simulink model "FOC_PMSM"  (R2021a)
settings: Solver=ode3  StartTime=0.0  StopTime=1  FixedStep=1e-6  RelTol=1e-3
InitFcn:
  | Td=1/5000;
  | Ld=0.0057;
  | Lq=0.0125;
  | r=1.2;
  | P=4;
  | Ld=0.0125;
  | Lq=0.0057;
  | PhiPM=0.123;
  | Vdc=700;
  | B=0;
  | J=0.0027;
  | fs=5000;
libraries: pid_lib x7, spsThreePhaseSeriesRLCBranchLib x3, spsThreePhaseVIMeasurementLib x2, spsdq0toabcLib x2, autolibpmsminterior x1, spsDCVoltageSourceLib x1, spsGroundLib x1, spsSVPWMGenerator2LevelLib x1, spsUniversalBridgeLib x1, spsabctoAlphaBetaZeroLib x1, spspowerguiLib x1, simulink x1
settings Model: Creator=Mostafa  LastModifiedBy=Mostafa

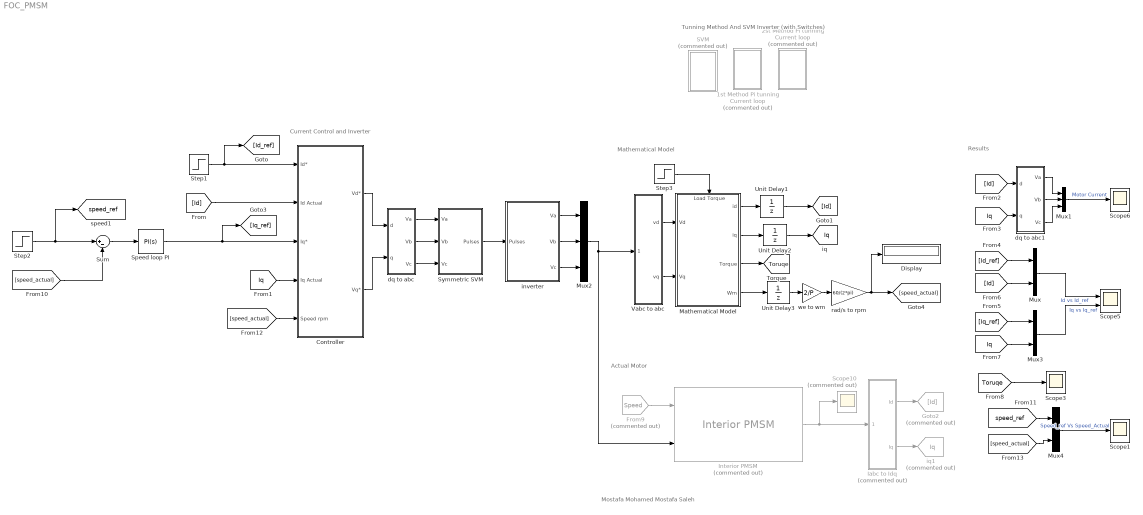
== system FOC_PMSM ==
  note: Tunning Method And SVM Inverter (with Switches)
  note: Current Control and Inverter
  note: Actual Motor
  note: Mathematical Model
  note: Results
  note: Mostafa Mohamed Mostafa Saleh
  1st Method Pi tunning Current loop : Subsystem  Commented=on
  2st Method Pi tunning Current loop : Subsystem  Commented=on
  Controller : Subsystem
  Display : Display
  From9 : From  Commented=on  GotoTag=Speed  TagVisibility=global
  Goto2 : Goto  Commented=on  GotoTag=Id
  Iabc to Idq : Subsystem  Commented=on
  Interior PMSM : autolibpmsminterior/Interior PMSM  Commented=on  port_config=Speed  sim_type=Continuous  Ts=0.001  P=2  Rs=1.2  Ldq=[0.125 0.057]  KConstText=Permanent flux linkage constant (lambda_pm):  lambda_pm=0.123  Ke=159.9771  mechanical=[0.0027, 4.924e-4, 0]  idq0=[0 0]  theta_init=0  omega_init=0  KConst=0.123  lambda_pm_calc=0.123  Kt=1.323  RefBlkName='autolibpmsminterior/Interior PMSM'  aMode=1
      settings: SourceProductBaseCode=PW,MT,VE,VP
  Mathematical Model : Subsystem
      settings: PortSchema="{\"entries\":[{\"content\":{\"sides\":[{\"content\":{\"connectorIds\":[\"In1\",\"In2\"]},\"type\":\"ConnectorPlacement.EquallySpacedRectSide\",\"uuid\":\"051f3cf9-9be1-4106-b38d-66cc7393fb99\"},{\"content\":{\"connectorIds\":[\"Out1\",\"Out2\",\"Out3\",\"Out4\"],\"side\":\"RIGHT\"},\"type\":\"ConnectorPlacement.EquallySpacedRectSide\",\"uuid\":\"0ae6f8d8-defd-4982-a857-4d094ecd69f7\"},{\"content\":{\"connectorIds\":[\"In3\"],\"side\":\"TOP\"},\"type\":\"ConnectorPlacement.EquallySpacedRectSide\",\"uuid\":\"9e822861-0fa2-4e7e-872b-d3c49c871a81\"}]},\"type\":\"ConnectorPlacement.EquallySpacedConnector\",\"uuid\":\"055cbe4c-d848-4a6f-bb15-48a4c380dc2b\"}],\"packageUris\":[\"http://schema.mathworks.com/mf0/Connector/R2020b\"],\"version\":\"1.0\"}"
  Mux : Mux  Inputs=2
  Mux1 : Mux  Inputs=3
  Mux2 : Mux  Inputs=3
  Mux3 : Mux  Inputs=2
  Mux4 : Mux  Inputs=2
  SVM : Subsystem  Commented=on
  Scope1 : Scope
  Scope10 : Scope  Commented=on
  Scope3 : Scope
  Scope5 : Scope  NumInputPorts=2
  Scope6 : Scope
  Speed loop PI : pid_lib/PID Controller  Controller=PI  Form=Parallel  TimeDomain=Continuous-time  UseExternalTs=off  SampleTime=-1  IntegratorMethod=Forward Euler  FilterMethod=Forward Euler  ControllerParametersSource=internal  P=0.642857  I=76.5306  D=0  UseFilter=on  N=100  TunerSelectOption=Transfer Function Based (PID Tuner App)  ZeroCross=off  InitialConditionSource=internal  InitialConditionForIntegrator=0  InitialConditionForFilter=0  DifferentiatorICPrevScaledInput=0  ExternalReset=none  TrackingMode=off  Kt=1  LimitOutput=on  SatLimitsSource=internal  UpperSaturationLimit=20  LowerSaturationLimit=-20  LinearizeAsGain=off  AntiWindupMode=clamping  Kb=1  POutMin=[]  POutMax=[]  IOutMin=[]  IOutMax=[]  DOutMin=[]  DOutMax=[]  NOutMin=[]  NOutMax=[]  SumOutMin=[]  SumOutMax=[]  SaturationOutMin=[]  SaturationOutMax=[]  PParamMin=[]  PParamMax=[]  IParamMin=[]  IParamMax=[]  DParamMin=[]  DParamMax=[]  NParamMin=[]  NParamMax=[]  KbParamMin=[]  KbParamMax=[]  KtParamMin=[]  KtParamMax=[]  KbOutMin=[]  KbOutMax=[]  KtOutMin=[]  KtOutMax=[]  IntegratorOutMin=[]  IntegratorOutMax=[]  FilterOutMin=[]  FilterOutMax=[]  SumI1OutMin=[]  SumI1OutMax=[]  SumI2OutMin=[]  SumI2OutMax=[]  SumI3OutMin=[]  SumI3OutMax=[]  SumI4OutMin=[]  SumI4OutMax=[]  SumDOutMin=[]  SumDOutMax=[]  DifferentiatorOutMin=[]  DifferentiatorOutMax=[]  FilterDiffOutCoefMin=[]  FilterDiffOutCoefMax=[]  ReciprocalOutMin=[]  ReciprocalOutMax=[]  SumDenOutMin=[]  SumDenOutMax=[]  SumNumOutMin=[]  SumNumOutMax=[]  DivideOutMin=[]  DivideOutMax=[]  UdiffTsProdOutMin=[]  UdiffTsProdOutMax=[]  NTsProdOutMin=[]  NTsProdOutMax=[]  UintegralTsProdOutMin=[]  UintegralTsProdOutMax=[]  UngainTsProdOutMin=[]  UngainTsProdOutMax=[]  IntegratorContinuousStateAttributes=''  IntegratorStateMustResolveToSignalObject=off  IntegratorRTWStateStorageClass=Auto  FilterContinuousStateAttributes=''  FilterStateMustResolveToSignalObject=off  FilterRTWStateStorageClass=Auto  ParallelPVariant=InternalParameters  IdealPVariant=Disabled  IVariant=InternalParameters  DVariant=Disabled  IntegratorVariant=Continuous  SatVariant=Enabled  AWVariant=ContClampingParallel  PCopyVariant=Disabled  TRVariant=Disabled  FdbkBlocksVariant=Forward  IdealPFdbkVariant=Disabled  SatFdbkVariant=Disabled  DerivativeFilterVariant=Disabled  NVariant=Disabled  NCopyVariant=Disabled_SignalSpec  FilterICVariant=Disabled  IntegratorICVariant=InternalICs  ExternalResetVariant=Disabled  TRSumVariant=Passthrough  SumFdbkVariant=Disabled  SumVariant=Sum_PI  TsampFilterVariant=InternalTs  TsampNgainVariant=Passthrough  TsampIntegralVariant=Passthrough  ExternalSaturationOutDataTypeStr=Inherit: Same as second input
  Step1 : Step  Time=0.2  After=0  SampleTime=0
  Step2 : Step  Time=0.2  After=1000  SampleTime=0
  Step3 : Step  Time=0.6  After=5  SampleTime=0
  Sum : Sum  Inputs=|+-
  Symmetric SVM : Subsystem
  Unit Delay1 : UnitDelay  SampleTime=-1  HasFrameUpgradeWarning=on
  Unit Delay2 : UnitDelay  SampleTime=-1  HasFrameUpgradeWarning=on
  Unit Delay3 : UnitDelay  SampleTime=-1  HasFrameUpgradeWarning=on
  Vabc to abc : Subsystem
  dq to abc : Subsystem
  dq to abc1 : Subsystem
  inverter : Subsystem
  iq1 : Goto  Commented=on  GotoTag=Iq  TagVisibility=global
  rad/s to rpm : Gain  Gain=60/(2*pi)
  we to wm : Gain  Gain=2/P
  tag scope: Iq=global, Toruqe=global, speed_ref=global
  wires:
  [Id] -> dq to abc1/1(d)
  [Toruqe] -> Scope3/1
  [Iq_ref] -> Mux3/1
  [Id] -> Mux/2
  Mux/1 -> Scope5/1  "Id vs Id_ref"
  Mux3/1 -> Scope5/2  "Iq vs Iq_ref"
  [Iq] -> Mux3/2
  [Id_ref] -> Mux/1
  [Iq] -> dq to abc1/2(q)
  Unit Delay2/1 -> [Iq]
  Step3/1 -> Mathematical Model/3(Load Torque)
  Mathematical Model/4(Wm) -> Unit Delay3/1
  Mathematical Model/2(iq) -> Unit Delay2/1
  Vabc to abc/1(vd) -> Mathematical Model/1(Vd)
  Vabc to abc/2(vq) -> Mathematical Model/2(Vq)
  Mathematical Model/3(Torque) -> [Toruqe]
  Unit Delay1/1 -> [Id]
  Mathematical Model/1(id) -> Unit Delay1/1
  Iabc to Idq/1(Id) -> Goto2/1
  From9/1 -> Interior PMSM/1
  Iabc to Idq/2(Iq) -> iq1/1
  Interior PMSM/2 -> Iabc to Idq/1(Iabc), Scope10/1
  Mux2/1 -> Interior PMSM/2, Vabc to abc/1(Vabc)
  inverter/1(Va) -> Mux2/1
  inverter/2(Vb) -> Mux2/2
  inverter/3(Vc) -> Mux2/3
  [Iq] -> Controller/4("Iq Actual ")
  Speed loop PI/1 -> [Iq_ref], Controller/3(Iq*)
  Symmetric SVM/1(Pulses) -> inverter/1(Pulses)
  dq to abc/1(Va) -> Symmetric SVM/1(Va)
  Controller/2(Vq*) -> dq to abc/2(q)
  dq to abc/2(Vb) -> Symmetric SVM/2(Vb)
  Step1/1 -> Controller/1(Id*), [Id_ref]
  [Id] -> Controller/2("Id Actual ")
  Controller/1(Vd*) -> dq to abc/1(d)
  dq to abc/3(Vc) -> Symmetric SVM/3(Vc)
  dq to abc1/1(Va) -> Mux1/1
  dq to abc1/2(Vb) -> Mux1/2
  dq to abc1/3(Vc) -> Mux1/3
  Mux1/1 -> Scope6/1  "Motor Current"
  Step2/1 -> [speed_ref], Sum/1
  [speed_actual] -> Sum/2
  Sum/1 -> Speed loop PI/1
  [speed_actual] -> Controller/5(Speed rpm)
  we to wm/1 -> rad/s to rpm/1
  Unit Delay3/1 -> we to wm/1
  rad/s to rpm/1 -> [speed_actual], Display/1
  [speed_ref] -> Mux4/1
  [speed_actual] -> Mux4/2
  Mux4/1 -> Scope1/1  "Speed_ref Vs Speed_Actual"

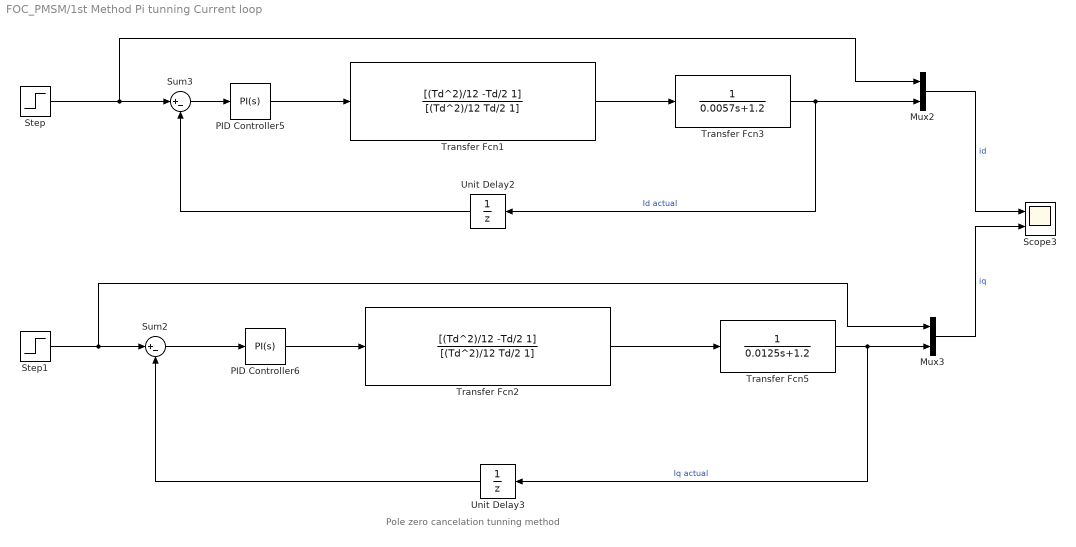
== system FOC_PMSM/1st Method Pi tunning Current loop ==
  note: Pole zero cancelation tunning method
  Mux2 : Mux  Inputs=2
  Mux3 : Mux  Inputs=2
  PID Controller5 : pid_lib/PID Controller  Controller=PI  Form=Parallel  TimeDomain=Continuous-time  UseExternalTs=off  SampleTime=-1  IntegratorMethod=Forward Euler  FilterMethod=Forward Euler  ControllerParametersSource=internal  P=9.405  I=1980  D=0  UseFilter=on  N=100  TunerSelectOption=Transfer Function Based (PID Tuner App)  InitialConditionSource=internal  InitialConditionForIntegrator=0  InitialConditionForFilter=0  DifferentiatorICPrevScaledInput=0  ExternalReset=none  TrackingMode=off  Kt=1  LimitOutput=off  SatLimitsSource=internal  UpperSaturationLimit=inf  LowerSaturationLimit=-inf  LinearizeAsGain=on  AntiWindupMode=clamping  Kb=1  POutMin=[]  POutMax=[]  IOutMin=[]  IOutMax=[]  DOutMin=[]  DOutMax=[]  NOutMin=[]  NOutMax=[]  SumOutMin=[]  SumOutMax=[]  SaturationOutMin=[]  SaturationOutMax=[]  PParamMin=[]  PParamMax=[]  IParamMin=[]  IParamMax=[]  DParamMin=[]  DParamMax=[]  NParamMin=[]  NParamMax=[]  KbParamMin=[]  KbParamMax=[]  KtParamMin=[]  KtParamMax=[]  KbOutMin=[]  KbOutMax=[]  KtOutMin=[]  KtOutMax=[]  IntegratorOutMin=[]  IntegratorOutMax=[]  FilterOutMin=[]  FilterOutMax=[]  SumI1OutMin=[]  SumI1OutMax=[]  SumI2OutMin=[]  SumI2OutMax=[]  SumI3OutMin=[]  SumI3OutMax=[]  SumI4OutMin=[]  SumI4OutMax=[]  SumDOutMin=[]  SumDOutMax=[]  DifferentiatorOutMin=[]  DifferentiatorOutMax=[]  FilterDiffOutCoefMin=[]  FilterDiffOutCoefMax=[]  ReciprocalOutMin=[]  ReciprocalOutMax=[]  SumDenOutMin=[]  SumDenOutMax=[]  SumNumOutMin=[]  SumNumOutMax=[]  DivideOutMin=[]  DivideOutMax=[]  UdiffTsProdOutMin=[]  UdiffTsProdOutMax=[]  NTsProdOutMin=[]  NTsProdOutMax=[]  UintegralTsProdOutMin=[]  UintegralTsProdOutMax=[]  UngainTsProdOutMin=[]  UngainTsProdOutMax=[]  IntegratorContinuousStateAttributes=''  IntegratorStateMustResolveToSignalObject=off  IntegratorRTWStateStorageClass=Auto  FilterContinuousStateAttributes=''  FilterStateMustResolveToSignalObject=off  FilterRTWStateStorageClass=Auto  ParallelPVariant=InternalParameters  IdealPVariant=Disabled  IVariant=InternalParameters  DVariant=Disabled  IntegratorVariant=Continuous  SatVariant=Disabled  AWVariant=Passthrough  PCopyVariant=Disabled  TRVariant=Disabled  FdbkBlocksVariant=Forward  IdealPFdbkVariant=Disabled  SatFdbkVariant=Disabled  DerivativeFilterVariant=Disabled  NVariant=Disabled  NCopyVariant=Disabled_SignalSpec  FilterICVariant=Disabled  IntegratorICVariant=InternalICs  ExternalResetVariant=Disabled  TRSumVariant=Passthrough  SumFdbkVariant=Disabled  SumVariant=Sum_PI  TsampFilterVariant=InternalTs  TsampNgainVariant=Passthrough  TsampIntegralVariant=Passthrough  ExternalSaturationOutDataTypeStr=Inherit: Same as second input
  PID Controller6 : pid_lib/PID Controller  Controller=PI  Form=Parallel  TimeDomain=Continuous-time  UseExternalTs=off  SampleTime=-1  IntegratorMethod=Forward Euler  FilterMethod=Forward Euler  ControllerParametersSource=internal  P=20.625  I=1980  D=0  UseFilter=on  N=100  TunerSelectOption=Transfer Function Based (PID Tuner App)  ZeroCross=off  InitialConditionSource=internal  InitialConditionForIntegrator=0  InitialConditionForFilter=0  DifferentiatorICPrevScaledInput=0  ExternalReset=none  TrackingMode=off  Kt=1  LimitOutput=off  SatLimitsSource=internal  UpperSaturationLimit=inf  LowerSaturationLimit=-inf  LinearizeAsGain=on  AntiWindupMode=clamping  Kb=1  POutMin=[]  POutMax=[]  IOutMin=[]  IOutMax=[]  DOutMin=[]  DOutMax=[]  NOutMin=[]  NOutMax=[]  SumOutMin=[]  SumOutMax=[]  SaturationOutMin=[]  SaturationOutMax=[]  PParamMin=[]  PParamMax=[]  IParamMin=[]  IParamMax=[]  DParamMin=[]  DParamMax=[]  NParamMin=[]  NParamMax=[]  KbParamMin=[]  KbParamMax=[]  KtParamMin=[]  KtParamMax=[]  KbOutMin=[]  KbOutMax=[]  KtOutMin=[]  KtOutMax=[]  IntegratorOutMin=[]  IntegratorOutMax=[]  FilterOutMin=[]  FilterOutMax=[]  SumI1OutMin=[]  SumI1OutMax=[]  SumI2OutMin=[]  SumI2OutMax=[]  SumI3OutMin=[]  SumI3OutMax=[]  SumI4OutMin=[]  SumI4OutMax=[]  SumDOutMin=[]  SumDOutMax=[]  DifferentiatorOutMin=[]  DifferentiatorOutMax=[]  FilterDiffOutCoefMin=[]  FilterDiffOutCoefMax=[]  ReciprocalOutMin=[]  ReciprocalOutMax=[]  SumDenOutMin=[]  SumDenOutMax=[]  SumNumOutMin=[]  SumNumOutMax=[]  DivideOutMin=[]  DivideOutMax=[]  UdiffTsProdOutMin=[]  UdiffTsProdOutMax=[]  NTsProdOutMin=[]  NTsProdOutMax=[]  UintegralTsProdOutMin=[]  UintegralTsProdOutMax=[]  UngainTsProdOutMin=[]  UngainTsProdOutMax=[]  IntegratorContinuousStateAttributes=''  IntegratorStateMustResolveToSignalObject=off  IntegratorRTWStateStorageClass=Auto  FilterContinuousStateAttributes=''  FilterStateMustResolveToSignalObject=off  FilterRTWStateStorageClass=Auto  ParallelPVariant=InternalParameters  IdealPVariant=Disabled  IVariant=InternalParameters  DVariant=Disabled  IntegratorVariant=Continuous  SatVariant=Disabled  AWVariant=Passthrough  PCopyVariant=Disabled  TRVariant=Disabled  FdbkBlocksVariant=Forward  IdealPFdbkVariant=Disabled  SatFdbkVariant=Disabled  DerivativeFilterVariant=Disabled  NVariant=Disabled  NCopyVariant=Disabled_SignalSpec  FilterICVariant=Disabled  IntegratorICVariant=InternalICs  ExternalResetVariant=Disabled  TRSumVariant=Passthrough  SumFdbkVariant=Disabled  SumVariant=Sum_PI  TsampFilterVariant=InternalTs  TsampNgainVariant=Passthrough  TsampIntegralVariant=Passthrough  ExternalSaturationOutDataTypeStr=Inherit: Same as second input
  Scope3 : Scope  NumInputPorts=2
  Step : Step  Time=0.1  SampleTime=0
  Step1 : Step  Time=0.1  SampleTime=0
  Sum2 : Sum  Inputs=|+-
  Sum3 : Sum  Inputs=|+-
  Transfer Fcn1 : TransferFcn  Numerator=[(Td^2)/12 -Td/2 1]  Denominator=[(Td^2)/12 Td/2 1]
  Transfer Fcn2 : TransferFcn  Numerator=[(Td^2)/12 -Td/2 1]  Denominator=[(Td^2)/12 Td/2 1]
  Transfer Fcn3 : TransferFcn  Denominator=[0.0057 1.2]
  Transfer Fcn5 : TransferFcn  Denominator=[0.0125 1.2]
  Unit Delay2 : UnitDelay  SampleTime=-1  HasFrameUpgradeWarning=on
  Unit Delay3 : UnitDelay  SampleTime=-1  HasFrameUpgradeWarning=on
  wires:
  Sum2/1 -> PID Controller6/1
  Unit Delay2/1 -> Sum3/2
  Transfer Fcn3/1 -> Mux2/2, Unit Delay2/1  "Id actual"
  Unit Delay3/1 -> Sum2/2
  Mux3/1 -> Scope3/2  "iq"
  Mux2/1 -> Scope3/1  "id"
  Transfer Fcn1/1 -> Transfer Fcn3/1
  Step/1 -> Sum3/1, Mux2/1
  PID Controller5/1 -> Transfer Fcn1/1
  Step1/1 -> Sum2/1, Mux3/1
  Transfer Fcn5/1 -> Mux3/2, Unit Delay3/1  "Iq actual"
  Sum3/1 -> PID Controller5/1
  PID Controller6/1 -> Transfer Fcn2/1
  Transfer Fcn2/1 -> Transfer Fcn5/1

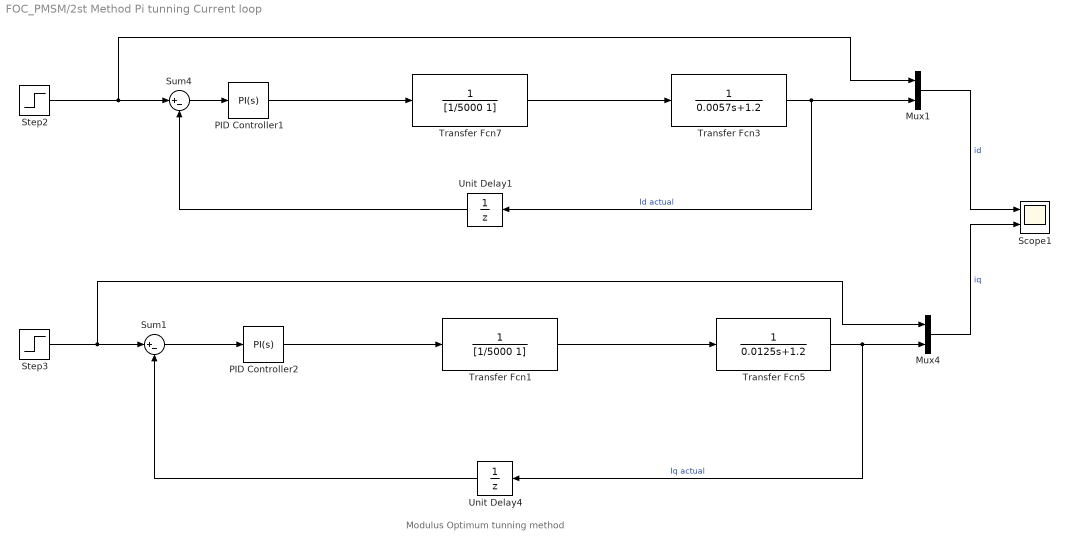
== system FOC_PMSM/2st Method Pi tunning Current loop ==
  note: Modulus Optimum tunning method
  Mux1 : Mux  Inputs=2
  Mux4 : Mux  Inputs=2
  PID Controller1 : pid_lib/PID Controller  Controller=PI  Form=Parallel  TimeDomain=Continuous-time  UseExternalTs=off  SampleTime=-1  IntegratorMethod=Forward Euler  FilterMethod=Forward Euler  ControllerParametersSource=internal  P=14.25  I=3000  D=0  UseFilter=on  N=100  TunerSelectOption=Transfer Function Based (PID Tuner App)  InitialConditionSource=internal  InitialConditionForIntegrator=0  InitialConditionForFilter=0  DifferentiatorICPrevScaledInput=0  ExternalReset=none  TrackingMode=off  Kt=1  LimitOutput=off  SatLimitsSource=internal  UpperSaturationLimit=inf  LowerSaturationLimit=-inf  LinearizeAsGain=on  AntiWindupMode=clamping  Kb=1  POutMin=[]  POutMax=[]  IOutMin=[]  IOutMax=[]  DOutMin=[]  DOutMax=[]  NOutMin=[]  NOutMax=[]  SumOutMin=[]  SumOutMax=[]  SaturationOutMin=[]  SaturationOutMax=[]  PParamMin=[]  PParamMax=[]  IParamMin=[]  IParamMax=[]  DParamMin=[]  DParamMax=[]  NParamMin=[]  NParamMax=[]  KbParamMin=[]  KbParamMax=[]  KtParamMin=[]  KtParamMax=[]  KbOutMin=[]  KbOutMax=[]  KtOutMin=[]  KtOutMax=[]  IntegratorOutMin=[]  IntegratorOutMax=[]  FilterOutMin=[]  FilterOutMax=[]  SumI1OutMin=[]  SumI1OutMax=[]  SumI2OutMin=[]  SumI2OutMax=[]  SumI3OutMin=[]  SumI3OutMax=[]  SumI4OutMin=[]  SumI4OutMax=[]  SumDOutMin=[]  SumDOutMax=[]  DifferentiatorOutMin=[]  DifferentiatorOutMax=[]  FilterDiffOutCoefMin=[]  FilterDiffOutCoefMax=[]  ReciprocalOutMin=[]  ReciprocalOutMax=[]  SumDenOutMin=[]  SumDenOutMax=[]  SumNumOutMin=[]  SumNumOutMax=[]  DivideOutMin=[]  DivideOutMax=[]  UdiffTsProdOutMin=[]  UdiffTsProdOutMax=[]  NTsProdOutMin=[]  NTsProdOutMax=[]  UintegralTsProdOutMin=[]  UintegralTsProdOutMax=[]  UngainTsProdOutMin=[]  UngainTsProdOutMax=[]  IntegratorContinuousStateAttributes=''  IntegratorStateMustResolveToSignalObject=off  IntegratorRTWStateStorageClass=Auto  FilterContinuousStateAttributes=''  FilterStateMustResolveToSignalObject=off  FilterRTWStateStorageClass=Auto  ParallelPVariant=InternalParameters  IdealPVariant=Disabled  IVariant=InternalParameters  DVariant=Disabled  IntegratorVariant=Continuous  SatVariant=Disabled  AWVariant=Passthrough  PCopyVariant=Disabled  TRVariant=Disabled  FdbkBlocksVariant=Forward  IdealPFdbkVariant=Disabled  SatFdbkVariant=Disabled  DerivativeFilterVariant=Disabled  NVariant=Disabled  NCopyVariant=Disabled_SignalSpec  FilterICVariant=Disabled  IntegratorICVariant=InternalICs  ExternalResetVariant=Disabled  TRSumVariant=Passthrough  SumFdbkVariant=Disabled  SumVariant=Sum_PI  TsampFilterVariant=InternalTs  TsampNgainVariant=Passthrough  TsampIntegralVariant=Passthrough  ExternalSaturationOutDataTypeStr=Inherit: Same as second input
  PID Controller2 : pid_lib/PID Controller  Controller=PI  Form=Parallel  TimeDomain=Continuous-time  UseExternalTs=off  SampleTime=-1  IntegratorMethod=Forward Euler  FilterMethod=Forward Euler  ControllerParametersSource=internal  P=31.25  I=3000  D=0  UseFilter=on  N=100  TunerSelectOption=Transfer Function Based (PID Tuner App)  ZeroCross=off  InitialConditionSource=internal  InitialConditionForIntegrator=0  InitialConditionForFilter=0  DifferentiatorICPrevScaledInput=0  ExternalReset=none  TrackingMode=off  Kt=1  LimitOutput=off  SatLimitsSource=internal  UpperSaturationLimit=inf  LowerSaturationLimit=-inf  LinearizeAsGain=on  AntiWindupMode=clamping  Kb=1  POutMin=[]  POutMax=[]  IOutMin=[]  IOutMax=[]  DOutMin=[]  DOutMax=[]  NOutMin=[]  NOutMax=[]  SumOutMin=[]  SumOutMax=[]  SaturationOutMin=[]  SaturationOutMax=[]  PParamMin=[]  PParamMax=[]  IParamMin=[]  IParamMax=[]  DParamMin=[]  DParamMax=[]  NParamMin=[]  NParamMax=[]  KbParamMin=[]  KbParamMax=[]  KtParamMin=[]  KtParamMax=[]  KbOutMin=[]  KbOutMax=[]  KtOutMin=[]  KtOutMax=[]  IntegratorOutMin=[]  IntegratorOutMax=[]  FilterOutMin=[]  FilterOutMax=[]  SumI1OutMin=[]  SumI1OutMax=[]  SumI2OutMin=[]  SumI2OutMax=[]  SumI3OutMin=[]  SumI3OutMax=[]  SumI4OutMin=[]  SumI4OutMax=[]  SumDOutMin=[]  SumDOutMax=[]  DifferentiatorOutMin=[]  DifferentiatorOutMax=[]  FilterDiffOutCoefMin=[]  FilterDiffOutCoefMax=[]  ReciprocalOutMin=[]  ReciprocalOutMax=[]  SumDenOutMin=[]  SumDenOutMax=[]  SumNumOutMin=[]  SumNumOutMax=[]  DivideOutMin=[]  DivideOutMax=[]  UdiffTsProdOutMin=[]  UdiffTsProdOutMax=[]  NTsProdOutMin=[]  NTsProdOutMax=[]  UintegralTsProdOutMin=[]  UintegralTsProdOutMax=[]  UngainTsProdOutMin=[]  UngainTsProdOutMax=[]  IntegratorContinuousStateAttributes=''  IntegratorStateMustResolveToSignalObject=off  IntegratorRTWStateStorageClass=Auto  FilterContinuousStateAttributes=''  FilterStateMustResolveToSignalObject=off  FilterRTWStateStorageClass=Auto  ParallelPVariant=InternalParameters  IdealPVariant=Disabled  IVariant=InternalParameters  DVariant=Disabled  IntegratorVariant=Continuous  SatVariant=Disabled  AWVariant=Passthrough  PCopyVariant=Disabled  TRVariant=Disabled  FdbkBlocksVariant=Forward  IdealPFdbkVariant=Disabled  SatFdbkVariant=Disabled  DerivativeFilterVariant=Disabled  NVariant=Disabled  NCopyVariant=Disabled_SignalSpec  FilterICVariant=Disabled  IntegratorICVariant=InternalICs  ExternalResetVariant=Disabled  TRSumVariant=Passthrough  SumFdbkVariant=Disabled  SumVariant=Sum_PI  TsampFilterVariant=InternalTs  TsampNgainVariant=Passthrough  TsampIntegralVariant=Passthrough  ExternalSaturationOutDataTypeStr=Inherit: Same as second input
  Scope1 : Scope  NumInputPorts=2
  Step2 : Step  Time=0.1  SampleTime=0
  Step3 : Step  Time=0.1  SampleTime=0
  Sum1 : Sum  Inputs=|+-
  Sum4 : Sum  Inputs=|+-
  Transfer Fcn1 : TransferFcn  Denominator=[1/5000 1]
  Transfer Fcn3 : TransferFcn  Denominator=[0.0057 1.2]
  Transfer Fcn5 : TransferFcn  Denominator=[0.0125 1.2]
  Transfer Fcn7 : TransferFcn  Denominator=[1/5000 1]
  Unit Delay1 : UnitDelay  SampleTime=-1  HasFrameUpgradeWarning=on
  Unit Delay4 : UnitDelay  SampleTime=-1  HasFrameUpgradeWarning=on
  wires:
  Transfer Fcn7/1 -> Transfer Fcn3/1
  Sum1/1 -> PID Controller2/1
  Unit Delay4/1 -> Sum1/2
  Unit Delay1/1 -> Sum4/2
  Mux4/1 -> Scope1/2  "iq"
  Transfer Fcn3/1 -> Unit Delay1/1, Mux1/2  "Id actual"
  Transfer Fcn1/1 -> Transfer Fcn5/1
  Transfer Fcn5/1 -> Unit Delay4/1, Mux4/2  "Iq actual"
  Mux1/1 -> Scope1/1  "id"
  Sum4/1 -> PID Controller1/1
  PID Controller1/1 -> Transfer Fcn7/1
  PID Controller2/1 -> Transfer Fcn1/1
  Step2/1 -> Mux1/1, Sum4/1
  Step3/1 -> Mux4/1, Sum1/1

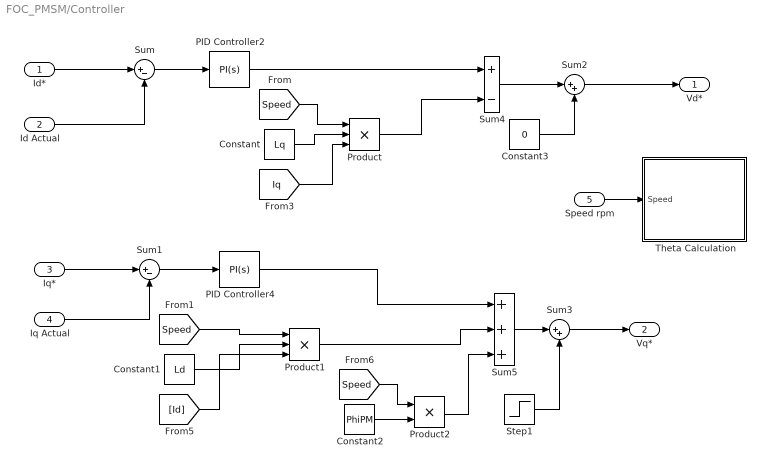
== system FOC_PMSM/Controller ==
  Id* : Inport
  "Id Actual " : Inport  Port=2
  Iq* : Inport  Port=3
  "Iq Actual " : Inport  Port=4
  Speed rpm : Inport  Port=5
  Constant : Constant  Value=Lq
  Constant1 : Constant  Value=Ld
  Constant2 : Constant  Value=PhiPM
  Constant3 : Constant  Value=0
  PID Controller2 : pid_lib/PID Controller  Controller=PI  Form=Parallel  TimeDomain=Continuous-time  UseExternalTs=off  SampleTime=-1  IntegratorMethod=Forward Euler  FilterMethod=Forward Euler  ControllerParametersSource=internal  P=14.25  I=3000  D=0  UseFilter=on  N=100  TunerSelectOption=Transfer Function Based (PID Tuner App)  ZeroCross=off  InitialConditionSource=internal  InitialConditionForIntegrator=0  InitialConditionForFilter=0  DifferentiatorICPrevScaledInput=0  ExternalReset=none  TrackingMode=off  Kt=1  LimitOutput=on  SatLimitsSource=internal  UpperSaturationLimit=Vdc/sqrt(3)  LowerSaturationLimit=-Vdc/sqrt(3)  LinearizeAsGain=off  AntiWindupMode=clamping  Kb=1  POutMin=[]  POutMax=[]  IOutMin=[]  IOutMax=[]  DOutMin=[]  DOutMax=[]  NOutMin=[]  NOutMax=[]  SumOutMin=[]  SumOutMax=[]  SaturationOutMin=[]  SaturationOutMax=[]  PParamMin=[]  PParamMax=[]  IParamMin=[]  IParamMax=[]  DParamMin=[]  DParamMax=[]  NParamMin=[]  NParamMax=[]  KbParamMin=[]  KbParamMax=[]  KtParamMin=[]  KtParamMax=[]  KbOutMin=[]  KbOutMax=[]  KtOutMin=[]  KtOutMax=[]  IntegratorOutMin=[]  IntegratorOutMax=[]  FilterOutMin=[]  FilterOutMax=[]  SumI1OutMin=[]  SumI1OutMax=[]  SumI2OutMin=[]  SumI2OutMax=[]  SumI3OutMin=[]  SumI3OutMax=[]  SumI4OutMin=[]  SumI4OutMax=[]  SumDOutMin=[]  SumDOutMax=[]  DifferentiatorOutMin=[]  DifferentiatorOutMax=[]  FilterDiffOutCoefMin=[]  FilterDiffOutCoefMax=[]  ReciprocalOutMin=[]  ReciprocalOutMax=[]  SumDenOutMin=[]  SumDenOutMax=[]  SumNumOutMin=[]  SumNumOutMax=[]  DivideOutMin=[]  DivideOutMax=[]  UdiffTsProdOutMin=[]  UdiffTsProdOutMax=[]  NTsProdOutMin=[]  NTsProdOutMax=[]  UintegralTsProdOutMin=[]  UintegralTsProdOutMax=[]  UngainTsProdOutMin=[]  UngainTsProdOutMax=[]  IntegratorContinuousStateAttributes=''  IntegratorStateMustResolveToSignalObject=off  IntegratorRTWStateStorageClass=Auto  FilterContinuousStateAttributes=''  FilterStateMustResolveToSignalObject=off  FilterRTWStateStorageClass=Auto  ParallelPVariant=InternalParameters  IdealPVariant=Disabled  IVariant=InternalParameters  DVariant=Disabled  IntegratorVariant=Continuous  SatVariant=Enabled  AWVariant=ContClampingParallel  PCopyVariant=Disabled  TRVariant=Disabled  FdbkBlocksVariant=Forward  IdealPFdbkVariant=Disabled  SatFdbkVariant=Disabled  DerivativeFilterVariant=Disabled  NVariant=Disabled  NCopyVariant=Disabled_SignalSpec  FilterICVariant=Disabled  IntegratorICVariant=InternalICs  ExternalResetVariant=Disabled  TRSumVariant=Passthrough  SumFdbkVariant=Disabled  SumVariant=Sum_PI  TsampFilterVariant=InternalTs  TsampNgainVariant=Passthrough  TsampIntegralVariant=Passthrough  ExternalSaturationOutDataTypeStr=Inherit: Same as second input
  PID Controller4 : pid_lib/PID Controller  Controller=PI  Form=Parallel  TimeDomain=Continuous-time  UseExternalTs=off  SampleTime=-1  IntegratorMethod=Forward Euler  FilterMethod=Forward Euler  ControllerParametersSource=internal  P=31.25  I=3000  D=0  UseFilter=on  N=100  TunerSelectOption=Transfer Function Based (PID Tuner App)  ZeroCross=off  InitialConditionSource=internal  InitialConditionForIntegrator=0  InitialConditionForFilter=0  DifferentiatorICPrevScaledInput=0  ExternalReset=none  TrackingMode=off  Kt=1  LimitOutput=on  SatLimitsSource=internal  UpperSaturationLimit=Vdc/sqrt(3)  LowerSaturationLimit=-Vdc/sqrt(3)  LinearizeAsGain=off  AntiWindupMode=clamping  Kb=1  POutMin=[]  POutMax=[]  IOutMin=[]  IOutMax=[]  DOutMin=[]  DOutMax=[]  NOutMin=[]  NOutMax=[]  SumOutMin=[]  SumOutMax=[]  SaturationOutMin=[]  SaturationOutMax=[]  PParamMin=[]  PParamMax=[]  IParamMin=[]  IParamMax=[]  DParamMin=[]  DParamMax=[]  NParamMin=[]  NParamMax=[]  KbParamMin=[]  KbParamMax=[]  KtParamMin=[]  KtParamMax=[]  KbOutMin=[]  KbOutMax=[]  KtOutMin=[]  KtOutMax=[]  IntegratorOutMin=[]  IntegratorOutMax=[]  FilterOutMin=[]  FilterOutMax=[]  SumI1OutMin=[]  SumI1OutMax=[]  SumI2OutMin=[]  SumI2OutMax=[]  SumI3OutMin=[]  SumI3OutMax=[]  SumI4OutMin=[]  SumI4OutMax=[]  SumDOutMin=[]  SumDOutMax=[]  DifferentiatorOutMin=[]  DifferentiatorOutMax=[]  FilterDiffOutCoefMin=[]  FilterDiffOutCoefMax=[]  ReciprocalOutMin=[]  ReciprocalOutMax=[]  SumDenOutMin=[]  SumDenOutMax=[]  SumNumOutMin=[]  SumNumOutMax=[]  DivideOutMin=[]  DivideOutMax=[]  UdiffTsProdOutMin=[]  UdiffTsProdOutMax=[]  NTsProdOutMin=[]  NTsProdOutMax=[]  UintegralTsProdOutMin=[]  UintegralTsProdOutMax=[]  UngainTsProdOutMin=[]  UngainTsProdOutMax=[]  IntegratorContinuousStateAttributes=''  IntegratorStateMustResolveToSignalObject=off  IntegratorRTWStateStorageClass=Auto  FilterContinuousStateAttributes=''  FilterStateMustResolveToSignalObject=off  FilterRTWStateStorageClass=Auto  ParallelPVariant=InternalParameters  IdealPVariant=Disabled  IVariant=InternalParameters  DVariant=Disabled  IntegratorVariant=Continuous  SatVariant=Enabled  AWVariant=ContClampingParallel  PCopyVariant=Disabled  TRVariant=Disabled  FdbkBlocksVariant=Forward  IdealPFdbkVariant=Disabled  SatFdbkVariant=Disabled  DerivativeFilterVariant=Disabled  NVariant=Disabled  NCopyVariant=Disabled_SignalSpec  FilterICVariant=Disabled  IntegratorICVariant=InternalICs  ExternalResetVariant=Disabled  TRSumVariant=Passthrough  SumFdbkVariant=Disabled  SumVariant=Sum_PI  TsampFilterVariant=InternalTs  TsampNgainVariant=Passthrough  TsampIntegralVariant=Passthrough  ExternalSaturationOutDataTypeStr=Inherit: Same as second input
  Product : Product  Inputs=3
  Product1 : Product  Inputs=3
  Product2 : Product
  Step1 : Step  Time=0.3  After=0  SampleTime=0
  Sum : Sum  Inputs=|+-
  Sum1 : Sum  Inputs=|+-
  Sum2 : Sum  Inputs=|++
  Sum3 : Sum  Inputs=|++
  Sum4 : Sum  Inputs=+-
  Sum5 : Sum  Inputs=+++
  Theta Calculation : Subsystem
  Vd* : Outport
  Vq* : Outport  Port=2
  wires:
  "Id Actual "/1 -> Sum/2
  Product/1 -> Sum4/2
  Id*/1 -> Sum/1
  Speed rpm/1 -> Theta Calculation/1(Speed)
  Sum/1 -> PID Controller2/1
  Sum1/1 -> PID Controller4/1
  [Speed] -> Product2/1
  Constant1/1 -> Product1/2
  [Speed] -> Product1/1
  [Speed] -> Product/1
  "Iq Actual "/1 -> Sum1/2
  Constant2/1 -> Product2/2
  Constant/1 -> Product/2
  Product1/1 -> Sum5/2
  Product2/1 -> Sum5/3
  Iq*/1 -> Sum1/1
  [Iq] -> Product/3
  [Id] -> Product1/3
  Sum4/1 -> Sum2/1
  Sum5/1 -> Sum3/1
  PID Controller2/1 -> Sum4/1
  PID Controller4/1 -> Sum5/1
  Sum2/1 -> Vd*/1
  Sum3/1 -> Vq*/1
  Constant3/1 -> Sum2/2
  Step1/1 -> Sum3/2

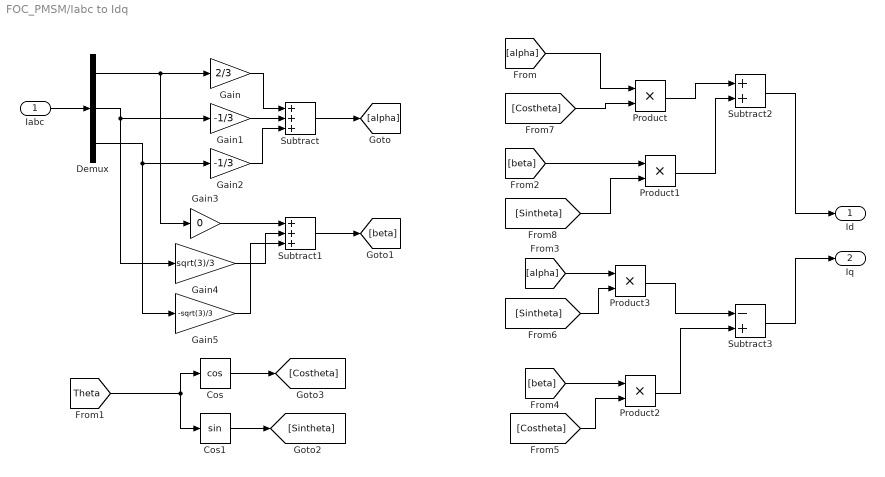
== system FOC_PMSM/Iabc to Idq ==
  Iabc : Inport
  Cos : Trigonometry  Operator=cos
  Cos1 : Trigonometry
  Demux : Demux  Outputs=3
  Gain : Gain  Gain=2/3
  Gain1 : Gain  Gain=-1/3
  Gain2 : Gain  Gain=-1/3
  Gain3 : Gain  Gain=0
  Gain4 : Gain  Gain=sqrt(3)/3
  Gain5 : Gain  Gain=-sqrt(3)/3
  Product{,1..3} (4 alike) : Product
  Subtract : Sum  Inputs=+++
  Subtract1 : Sum  Inputs=+++
  Subtract2 : Sum
  Subtract3 : Sum  Inputs=-+
  Id : Outport
  Iq : Outport  Port=2
  wires:
  [Sintheta] -> Product1/2
  Cos1/1 -> [Sintheta]
  [Sintheta] -> Product3/2
  [Costheta] -> Product/2
  Subtract3/1 -> Iq/1
  Subtract2/1 -> Id/1
  Product1/1 -> Subtract2/2
  [alpha] -> Product3/1
  Product3/1 -> Subtract3/1
  [beta] -> Product2/1
  Product2/1 -> Subtract3/2
  Cos/1 -> [Costheta]
  [beta] -> Product1/1
  Gain4/1 -> Subtract1/2
  Demux/3 -> Gain2/1, Gain5/1
  Gain5/1 -> Subtract1/3
  Gain2/1 -> Subtract/3
  [alpha] -> Product/1
  Demux/1 -> Gain3/1, Gain/1
  Gain/1 -> Subtract/1
  Subtract1/1 -> [beta]
  Product/1 -> Subtract2/1
  [Theta] -> Cos1/1, Cos/1
  [Costheta] -> Product2/2
  Gain1/1 -> Subtract/2
  Iabc/1 -> Demux/1
  Demux/2 -> Gain1/1, Gain4/1
  Gain3/1 -> Subtract1/1
  Subtract/1 -> [alpha]

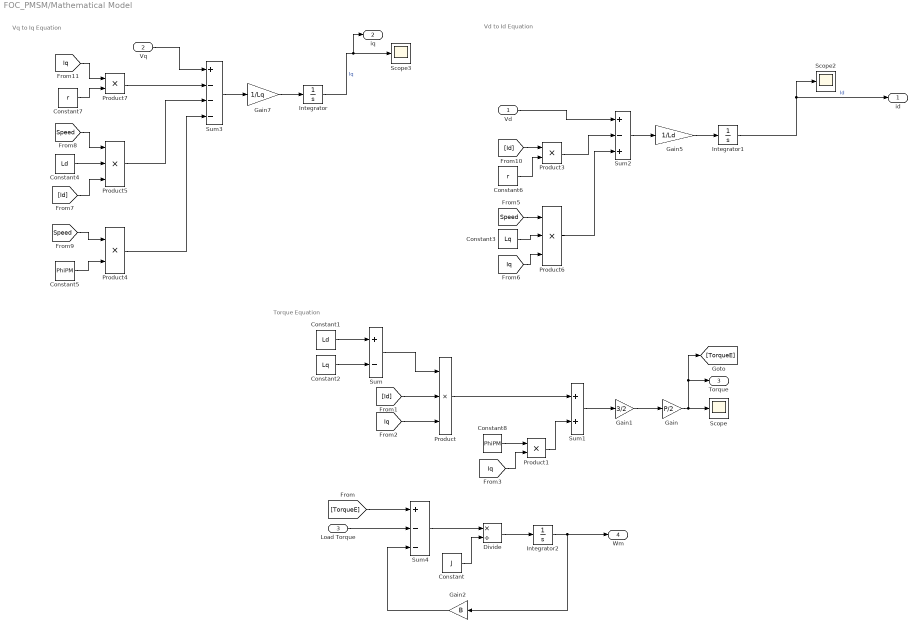
== system FOC_PMSM/Mathematical Model ==
  note: Vd to Id Equation
  note: Vq to Iq Equation
  note: Torque Equation
  Vd : Inport
  Vq : Inport  Port=2
  Load Torque : Inport  Port=3
  Constant : Constant  Value=J
  Constant1 : Constant  Value=Ld
  Constant2 : Constant  Value=Lq
  Constant3 : Constant  Value=Lq
  Constant4 : Constant  Value=Ld
  Constant5 : Constant  Value=PhiPM
  Constant6 : Constant  Value=r
  Constant7 : Constant  Value=r
  Constant8 : Constant  Value=PhiPM
  Divide : Product  Inputs=*/
  Gain : Gain  Gain=P/2
  Gain1 : Gain  Gain=3/2
  Gain2 : Gain  Gain=B
  Gain5 : Gain  Gain=1/Ld
  Gain7 : Gain  Gain=1/Lq
  Integrator : Integrator
  Integrator1 : Integrator
  Integrator2 : Integrator
  Product : Product  Inputs=3
  Product{1,3..4,7} (4 alike) : Product
  Product5 : Product  Inputs=3
  Product6 : Product  Inputs=3
  Scope : Scope
  Scope2 : Scope
  Scope3 : Scope
  Sum : Sum  Inputs=+-
  Sum1 : Sum
  Sum2 : Sum  Inputs=+-+
  Sum3 : Sum  Inputs=+---
  Sum4 : Sum  Inputs=+--
  id : Outport
  iq : Outport  Port=2
  Torque : Outport  Port=3
  Wm : Outport  Port=4
  wires:
  Constant8/1 -> Product1/1
  [Iq] -> Product/3
  Constant1/1 -> Sum/1
  Product1/1 -> Sum1/2
  [Id] -> Product/2
  [Iq] -> Product1/2
  Product/1 -> Sum1/1
  Constant2/1 -> Sum/2
  Sum/1 -> Product/1
  Sum1/1 -> Gain1/1
  Gain1/1 -> Gain/1
  Gain/1 -> [TorqueE], Torque/1, Scope/1
  [Id] -> Product5/3
  Constant5/1 -> Product4/2
  Constant4/1 -> Product5/2
  Sum3/1 -> Gain7/1
  Gain7/1 -> Integrator/1
  Product5/1 -> Sum3/3
  [Speed] -> Product4/1
  Constant7/1 -> Product7/2
  [Iq] -> Product7/1
  Product4/1 -> Sum3/4
  Product7/1 -> Sum3/2
  [Speed] -> Product5/1
  Vq/1 -> Sum3/1
  Integrator/1 -> iq/1, Scope3/1  "Iq"
  Product6/1 -> Sum2/3
  [Iq] -> Product6/3
  [Id] -> Product3/1
  Gain5/1 -> Integrator1/1
  Sum2/1 -> Gain5/1
  Vd/1 -> Sum2/1
  Constant6/1 -> Product3/2
  Product3/1 -> Sum2/2
  [Speed] -> Product6/1
  Constant3/1 -> Product6/2
  Integrator1/1 -> Scope2/1, id/1  "Id"
  [TorqueE] -> Sum4/1
  Load Torque/1 -> Sum4/2
  Sum4/1 -> Divide/1
  Constant/1 -> Divide/2
  Divide/1 -> Integrator2/1
  Integrator2/1 -> Gain2/1, Wm/1
  Gain2/1 -> Sum4/3

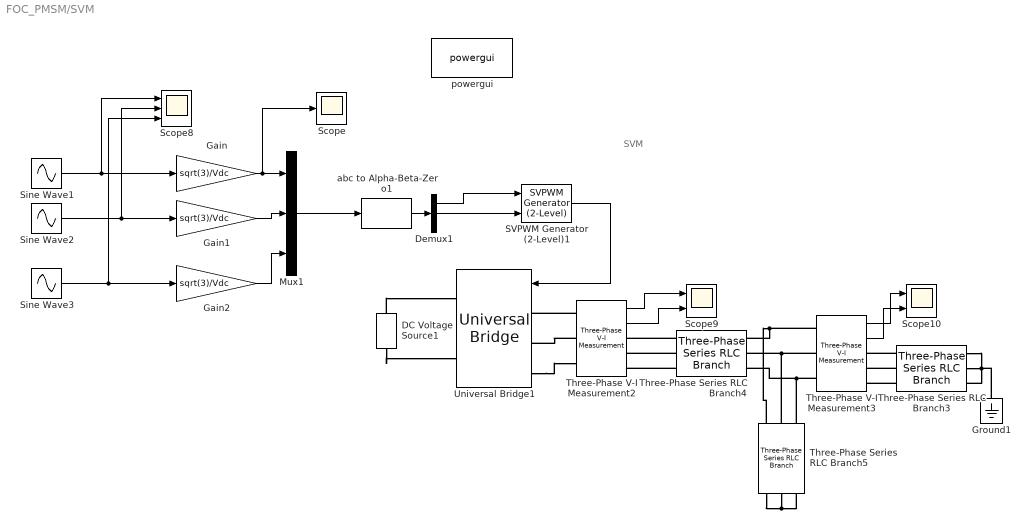
== system FOC_PMSM/SVM ==
  note: SVM
  DC Voltage Source1 : spsDCVoltageSourceLib/DC Voltage Source  Amplitude=Vdc  Measurements=None
  Demux1 : Demux  Outputs=3
  Gain : Gain  Gain=sqrt(3)/Vdc
  Gain1 : Gain  Gain=sqrt(3)/Vdc
  Gain2 : Gain  Gain=sqrt(3)/Vdc
  Ground1 : spsGroundLib/Ground  LConnTagsString=a
  Mux1 : Mux  Inputs=3
  SVPWM Generator (2-Level)1 : spsSVPWMGenerator2LevelLib/SVPWM Generator (2-Level)  InputType=alpha-beta components  SwitchingPattern=Pattern #1  Fc=5000  ParUref=[0.8 -30 50]  Ts=0
      settings: SourceProductBaseCode=PS
  Scope : Scope
  Scope10 : Scope  NumInputPorts=2
  Scope8 : Scope  NumInputPorts=3
  Scope9 : Scope  NumInputPorts=2
  Sine Wave1 : Sin  Amplitude=250  Frequency=100*pi  SampleTime=0
  Sine Wave2 : Sin  Amplitude=250  Frequency=100*pi  Phase=-2*pi/3  SampleTime=0
  Sine Wave3 : Sin  Amplitude=250  Frequency=100*pi  Phase=2*pi/3  SampleTime=0
  Three-Phase Series RLC Branch3 : spsThreePhaseSeriesRLCBranchLib/Three-Phase Series RLC Branch  LConnTagsString=A|B|C  RConnTagsString=A|B|C  BranchType=R  Resistance=10  Inductance=1e-3  Capacitance=1e-6  Measurements=None
  Three-Phase Series RLC Branch4 : spsThreePhaseSeriesRLCBranchLib/Three-Phase Series RLC Branch  LConnTagsString=A|B|C  RConnTagsString=A|B|C  BranchType=L  Resistance=1  Inductance=1e-3  Capacitance=1e-6  Measurements=None
  Three-Phase Series RLC Branch5 : spsThreePhaseSeriesRLCBranchLib/Three-Phase Series RLC Branch  LConnTagsString=A|B|C  RConnTagsString=A|B|C  BranchType=C  Resistance=1  Inductance=1e-3  Capacitance=100e-6  Measurements=None
  Three-Phase V-I Measurement2 : spsThreePhaseVIMeasurementLib/Three-Phase V-I Measurement  VoltageMeasurement=phase-to-ground  SetLabelV=off  LabelV=Vabc  Vpu=off  VpuLL=off  CurrentMeasurement=yes  SetLabelI=off  LabelI=Iabc  Ipu=off  Pbase=100e6  Vbase=500e3  OutputType=Complex  PhasorSimulation=off  PSBequivalent=0
  Three-Phase V-I Measurement3 : spsThreePhaseVIMeasurementLib/Three-Phase V-I Measurement  VoltageMeasurement=phase-to-ground  SetLabelV=off  LabelV=Vabc  Vpu=off  VpuLL=off  CurrentMeasurement=yes  SetLabelI=off  LabelI=Iabc  Ipu=off  Pbase=100e6  Vbase=500e3  OutputType=Complex  PhasorSimulation=off  PSBequivalent=0
  Universal Bridge1 : spsUniversalBridgeLib/Universal Bridge  Arms=3  SnubberResistance=1e5  SnubberCapacitance=inf  Device=IGBT / Diodes  Ron=1e-3  Lon=0  ForwardVoltages="[  0  0  ]"  ForwardVoltage=0  GTOparameters=[ 10e-6 , 20e-6 ]  IGBTparameters=[ 1e-6 , 2e-6 ]  Measurements=None  Measurements_2=None  converterType=Rectifier
  abc to Alpha-Beta-Zero1 : spsabctoAlphaBetaZeroLib/abc to Alpha-Beta-Zero
      settings: SourceProductBaseCode=PS
  powergui : spspowerguiLib/powergui  Priority=1  SimulationMode=Continuous  SampleTime=50e-6  frequency=60  Iterations=50  frequencyindice=0  Pbase=100e6  ErrMax=1e-4  UnitsV=kV  UnitsW=MW  buscounter=0  FunctionMessages=off  echomessages=off  EnableUseOfTLC=off  CurrentSourceSwitches=off  DisableSnubberDevices=off  DisableRonSwitches=off  DisableVfSwitches=off  DisplayEquations=off  AutomaticDiscreteSolvers=off  SolverType=Tustin/Backward Euler (TBE)  Interpol=off  ExternalGateDelay=off  methode=off  Ts=100  x0status=blocks  SPID=on  SwTol=0  HookPort=off  NonlinearTolerance=1e-4  nMaxIteration=100  ContinueOnMaxIteration=off  RestoreLinks=warning  ResistiveCurrentMeasurement=off  Frange=[0:2:500]  Ylog=off  Xlog=on  ShowGrid=off  save=off  variable=ZData  structure=0  ZoomFFT=off  StartTime=0.0  cycles=1  DisplayStyle=1  fundamental=60  FreqAxis=off  MaxFrequency=1000  frequencyindicesteady=1  RmsSteady=1  display=off
  wires:
  Gain2/1 -> Mux1/3
  Sine Wave3/1 -> Gain2/1, Scope8/3
  Three-Phase V-I Measurement2/1 -> Scope9/1
  Gain/1 -> Mux1/1, Scope/1
  Gain1/1 -> Mux1/2
  Three-Phase V-I Measurement3/1 -> Scope10/1
  Mux1/1 -> abc to Alpha-Beta-Zero1/1
  Demux1/2 -> SVPWM Generator (2-Level)1/2
  Demux1/1 -> SVPWM Generator (2-Level)1/1
  Three-Phase V-I Measurement2/2 -> Scope9/2
  SVPWM Generator (2-Level)1/1 -> Universal Bridge1/1
  Three-Phase V-I Measurement3/2 -> Scope10/2
  Sine Wave1/1 -> Gain/1, Scope8/1
  Sine Wave2/1 -> Gain1/1, Scope8/2
  abc to Alpha-Beta-Zero1/1 -> Demux1/1
  connections:
  Three-Phase Series RLC Branch4/RConn2 -- Three-Phase Series RLC Branch5/LConn2 -- Three-Phase V-I Measurement3/LConn2
  Three-Phase Series RLC Branch4/RConn3 -- Three-Phase Series RLC Branch5/LConn3 -- Three-Phase V-I Measurement3/LConn3
  Three-Phase Series RLC Branch3/RConn3 -- Three-Phase Series RLC Branch3/RConn2 -- Three-Phase Series RLC Branch3/RConn1 -- Ground1/LConn1
  Three-Phase Series RLC Branch5/RConn3 -- Three-Phase Series RLC Branch5/RConn2 -- Three-Phase Series RLC Branch5/RConn1
  Three-Phase Series RLC Branch4/RConn1 -- Three-Phase Series RLC Branch5/LConn1 -- Three-Phase V-I Measurement3/LConn1
  Universal Bridge1/LConn3 -- Three-Phase V-I Measurement2/LConn3
  DC Voltage Source1/LConn1 -- Universal Bridge1/RConn2
  Three-Phase Series RLC Branch3/LConn2 -- Three-Phase V-I Measurement3/RConn2
  DC Voltage Source1/RConn1 -- Universal Bridge1/RConn1
  Three-Phase V-I Measurement2/LConn2 -- Universal Bridge1/LConn2
  Three-Phase Series RLC Branch4/LConn2 -- Three-Phase V-I Measurement2/RConn2
  Three-Phase V-I Measurement2/LConn1 -- Universal Bridge1/LConn1
  Three-Phase Series RLC Branch3/LConn3 -- Three-Phase V-I Measurement3/RConn3
  Three-Phase Series RLC Branch4/LConn1 -- Three-Phase V-I Measurement2/RConn1
  Three-Phase Series RLC Branch4/LConn3 -- Three-Phase V-I Measurement2/RConn3
  Three-Phase Series RLC Branch3/LConn1 -- Three-Phase V-I Measurement3/RConn1

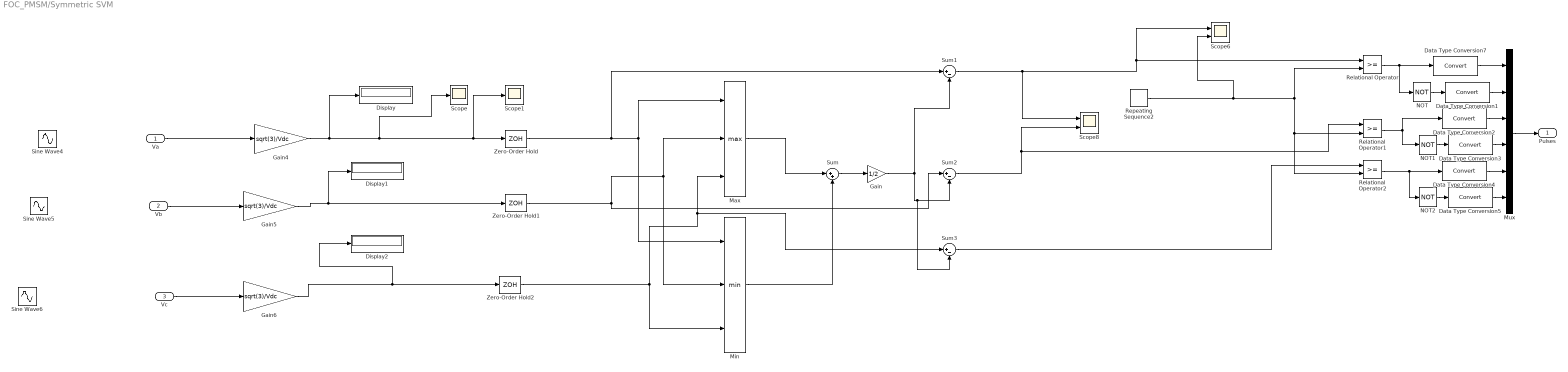
== system FOC_PMSM/Symmetric SVM ==
  Va : Inport
  Vb : Inport  Port=2
  Vc : Inport  Port=3
  Data Type Conversion{1..5,7} (6 alike) : DataTypeConversion
  Display : Display
  Display1 : Display
  Display2 : Display
  Gain : Gain  Gain=1/2
  Gain4 : Gain  Gain=sqrt(3)/Vdc
  Gain5 : Gain  Gain=sqrt(3)/Vdc
  Gain6 : Gain  Gain=sqrt(3)/Vdc
  Max : MinMax  Function=max  Inputs=3
  Min : MinMax  Inputs=3
  Mux : Mux  Inputs=6
  NOT : Logic  Operator=NOT  IconShape=distinctive  AllPortsSameDT=off  OutDataTypeStr=boolean
  NOT1 : Logic  Operator=NOT  IconShape=distinctive  AllPortsSameDT=off  OutDataTypeStr=boolean
  NOT2 : Logic  Operator=NOT  IconShape=distinctive  AllPortsSameDT=off  OutDataTypeStr=boolean
  Relational Operator : RelationalOperator  OutDataTypeStr=boolean  RndMeth=Simplest
  Relational Operator1 : RelationalOperator  OutDataTypeStr=boolean  RndMeth=Simplest
  Relational Operator2 : RelationalOperator  OutDataTypeStr=boolean  RndMeth=Simplest
  Repeating Sequence2 : simulink/Sources/Repeating Sequence  rep_seq_t=[0 1/(4*fs) 2/(4*fs) 3/(4*fs) 1/fs ]  rep_seq_y=[1 0 -1 0 1]
  Scope : Scope
  Scope1 : Scope
  Scope6 : Scope  NumInputPorts=2
  Scope8 : Scope  NumInputPorts=2
  Sine Wave4 : Sin  Amplitude=250  Frequency=100*pi  SampleTime=0
  Sine Wave5 : Sin  Amplitude=250  Frequency=100*pi  Phase=-2*pi/3  SampleTime=0
  Sine Wave6 : Sin  Amplitude=250  Frequency=100*pi  Phase=2*pi/3  SampleTime=0
  Sum : Sum  Inputs=|++
  Sum1 : Sum  Inputs=|+-
  Sum2 : Sum  Inputs=|+-
  Sum3 : Sum  Inputs=|+-
  Zero-Order Hold : ZeroOrderHold  SampleTime=1/fs
  Zero-Order Hold1 : ZeroOrderHold  SampleTime=1/fs
  Zero-Order Hold2 : ZeroOrderHold  SampleTime=1/fs
  Pulses : Outport
  wires:
  Vc/1 -> Gain6/1
  Vb/1 -> Gain5/1
  Va/1 -> Gain4/1
  Zero-Order Hold/1 -> Max/1, Min/1, Sum1/1
  Sum1/1 -> Scope8/1, Relational Operator/1, Scope6/1
  Sum2/1 -> Scope8/2, Relational Operator1/1
  Sum3/1 -> Relational Operator2/1
  Zero-Order Hold2/1 -> Min/3, Max/3, Sum3/1
  Min/1 -> Sum/2
  Max/1 -> Sum/1
  Gain/1 -> Sum1/2, Sum3/2, Sum2/2
  Zero-Order Hold1/1 -> Sum2/1, Max/2, Min/2
  Sum/1 -> Gain/1
  Repeating Sequence2/1 -> Relational Operator2/2, Relational Operator1/2, Relational Operator/2, Scope6/2
  Mux/1 -> Pulses/1
  Relational Operator/1 -> Data Type Conversion7/1, NOT/1
  NOT/1 -> Data Type Conversion1/1
  Relational Operator1/1 -> Data Type Conversion2/1, NOT1/1
  NOT1/1 -> Data Type Conversion3/1
  Relational Operator2/1 -> Data Type Conversion4/1, NOT2/1
  NOT2/1 -> Data Type Conversion5/1
  Data Type Conversion7/1 -> Mux/1
  Data Type Conversion1/1 -> Mux/2
  Data Type Conversion2/1 -> Mux/3
  Data Type Conversion3/1 -> Mux/4
  Data Type Conversion4/1 -> Mux/5
  Data Type Conversion5/1 -> Mux/6
  Gain4/1 -> Display/1, Scope1/1, Zero-Order Hold/1, Scope/1
  Gain5/1 -> Zero-Order Hold1/1, Display1/1
  Gain6/1 -> Zero-Order Hold2/1, Display2/1

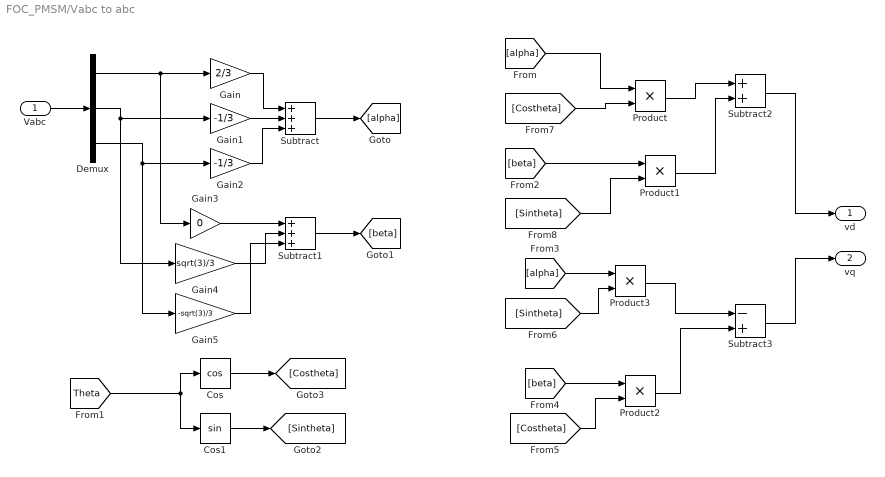
== system FOC_PMSM/Vabc to abc ==
  Vabc : Inport
  Cos : Trigonometry  Operator=cos
  Cos1 : Trigonometry
  Demux : Demux  Outputs=3
  Gain : Gain  Gain=2/3
  Gain1 : Gain  Gain=-1/3
  Gain2 : Gain  Gain=-1/3
  Gain3 : Gain  Gain=0
  Gain4 : Gain  Gain=sqrt(3)/3
  Gain5 : Gain  Gain=-sqrt(3)/3
  Product{,1..3} (4 alike) : Product
  Subtract : Sum  Inputs=+++
  Subtract1 : Sum  Inputs=+++
  Subtract2 : Sum
  Subtract3 : Sum  Inputs=-+
  vd : Outport
  vq : Outport  Port=2
  wires:
  Subtract/1 -> [alpha]
  Gain3/1 -> Subtract1/1
  Demux/2 -> Gain4/1, Gain1/1
  Vabc/1 -> Demux/1
  Gain1/1 -> Subtract/2
  [Costheta] -> Product2/2
  [Theta] -> Cos/1, Cos1/1
  Product/1 -> Subtract2/1
  Subtract1/1 -> [beta]
  Gain/1 -> Subtract/1
  Demux/1 -> Gain/1, Gain3/1
  [alpha] -> Product/1
  Gain2/1 -> Subtract/3
  Gain5/1 -> Subtract1/3
  Demux/3 -> Gain5/1, Gain2/1
  Gain4/1 -> Subtract1/2
  [beta] -> Product1/1
  Cos/1 -> [Costheta]
  Product2/1 -> Subtract3/2
  [beta] -> Product2/1
  Product3/1 -> Subtract3/1
  [alpha] -> Product3/1
  Product1/1 -> Subtract2/2
  Subtract2/1 -> vd/1
  Subtract3/1 -> vq/1
  [Costheta] -> Product/2
  [Sintheta] -> Product3/2
  Cos1/1 -> [Sintheta]
  [Sintheta] -> Product1/2

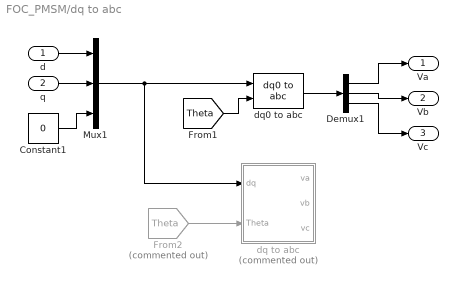
== system FOC_PMSM/dq to abc ==
  d : Inport
  q : Inport  Port=2
  Constant1 : Constant  Value=0
  Demux1 : Demux  Outputs=3
  From2 : From  Commented=on  GotoTag=Theta  TagVisibility=global
  Mux1 : Mux  Inputs=3
  dq to abc : Subsystem  Commented=on
  dq0 to abc : spsdq0toabcLib/dq0 to abc  Alignment=Aligned with phase A axis
  Va : Outport
  Vb : Outport  Port=2
  Vc : Outport  Port=3
  wires:
  dq0 to abc/1 -> Demux1/1
  Demux1/1 -> Va/1
  Mux1/1 -> dq to abc/1(dq), dq0 to abc/1
  q/1 -> Mux1/2
  Demux1/2 -> Vb/1
  d/1 -> Mux1/1
  Constant1/1 -> Mux1/3
  Demux1/3 -> Vc/1
  From2/1 -> dq to abc/2(Theta)
  [Theta] -> dq0 to abc/2

== system FOC_PMSM/dq to abc1 ==
  d : Inport
  q : Inport  Port=2
  Constant1 : Constant  Value=0
  Demux1 : Demux  Outputs=3
  Mux1 : Mux  Inputs=3
  dq0 to abc : spsdq0toabcLib/dq0 to abc  Alignment=Aligned with phase A axis
  Va : Outport
  Vb : Outport  Port=2
  Vc : Outport  Port=3
  wires:
  [Theta] -> dq0 to abc/2
  Demux1/3 -> Vc/1
  Constant1/1 -> Mux1/3
  d/1 -> Mux1/1
  Demux1/2 -> Vb/1
  q/1 -> Mux1/2
  Mux1/1 -> dq0 to abc/1
  Demux1/1 -> Va/1
  dq0 to abc/1 -> Demux1/1

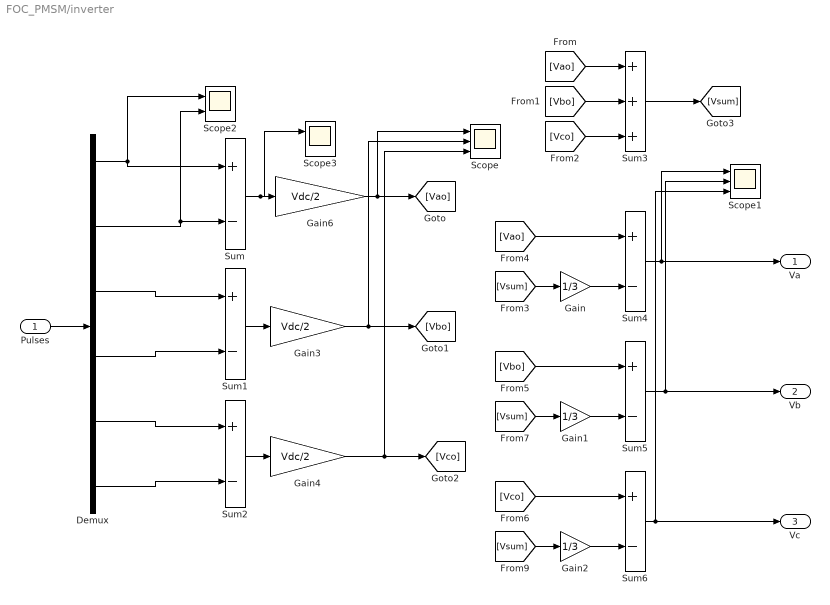
== system FOC_PMSM/inverter ==
  Pulses : Inport
  Demux : Demux  Outputs=6
  Gain : Gain  Gain=1/3
  Gain1 : Gain  Gain=1/3
  Gain2 : Gain  Gain=1/3
  Gain3 : Gain  Gain=Vdc/2
  Gain4 : Gain  Gain=Vdc/2
  Gain6 : Gain  Gain=Vdc/2
  Scope : Scope  NumInputPorts=3
  Scope1 : Scope  NumInputPorts=3
  Scope2 : Scope  NumInputPorts=2
  Scope3 : Scope  NumInputPorts=2
  Sum{,1..2,4..6} (6 alike) : Sum  Inputs=+-
  Sum3 : Sum  Inputs=+++
  Va : Outport
  Vb : Outport  Port=2
  Vc : Outport  Port=3
  wires:
  Sum2/1 -> Gain4/1
  Sum1/1 -> Gain3/1
  Sum/1 -> Scope3/1, Gain6/1
  Sum6/1 -> Scope1/3, Vc/1
  Sum5/1 -> Scope1/2, Vb/1
  Sum4/1 -> Scope1/1, Va/1
  Pulses/1 -> Demux/1
  Demux/1 -> Sum/1, Scope2/1
  Demux/2 -> Scope2/2, Sum/2
  Demux/3 -> Sum1/1
  Demux/4 -> Sum1/2
  Demux/5 -> Sum2/1
  Demux/6 -> Sum2/2
  [Vao] -> Sum3/1
  [Vbo] -> Sum3/2
  [Vco] -> Sum3/3
  Sum3/1 -> [Vsum]
  [Vsum] -> Gain/1
  [Vao] -> Sum4/1
  Gain/1 -> Sum4/2
  Gain1/1 -> Sum5/2
  [Vbo] -> Sum5/1
  [Vsum] -> Gain1/1
  [Vsum] -> Gain2/1
  [Vco] -> Sum6/1
  Gain2/1 -> Sum6/2
  Gain6/1 -> Scope/1, [Vao]
  Gain3/1 -> [Vbo], Scope/2
  Gain4/1 -> Scope/3, [Vco]

== system FOC_PMSM/Controller/Theta Calculation ==
  Speed : Inport
  Gain1 : Gain  Gain=P/2
  Gain2 : Gain  Gain=P/2
  Gain3 : Gain  Gain=2*pi/60
  Gain4 : Gain  Gain=2*pi/60
  Integrator : Integrator
  Scope2 : Scope
  tag scope: Speed=global, Theta=global
  wires:
  Speed/1 -> Gain4/1
  Gain2/1 -> [Speed]
  Integrator/1 -> [Theta], Scope2/1
  Gain1/1 -> Integrator/1
  Gain4/1 -> Gain1/1, Gain2/1

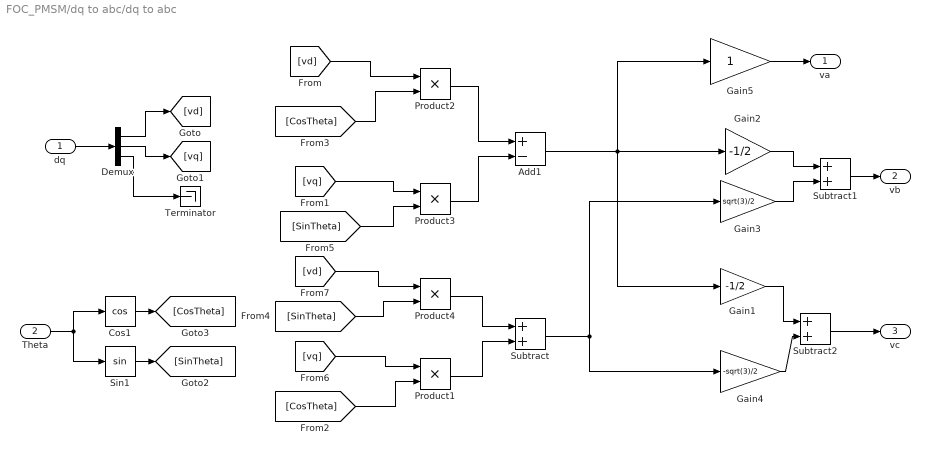
== system FOC_PMSM/dq to abc/dq to abc ==
  dq : Inport
  Theta : Inport  Port=2
  Add1 : Sum  Inputs=+-
  Cos1 : Trigonometry  Operator=cos
  Demux : Demux  Outputs=3
  Gain1 : Gain  Gain=-1/2
  Gain2 : Gain  Gain=-1/2
  Gain3 : Gain  Gain=sqrt(3)/2
  Gain4 : Gain  Gain=-sqrt(3)/2
  Gain5 : Gain
  Product{1..4} (4 alike) : Product
  Sin1 : Trigonometry
  Subtract : Sum
  Subtract1 : Sum
  Subtract2 : Sum
  Terminator : Terminator
  va : Outport
  vb : Outport  Port=2
  vc : Outport  Port=3
  wires:
  Product3/1 -> Add1/2
  Product1/1 -> Subtract/2
  Product2/1 -> Add1/1
  Product4/1 -> Subtract/1
  [vq] -> Product3/1
  [vd] -> Product2/1
  Subtract1/1 -> vb/1
  Gain5/1 -> va/1
  Subtract/1 -> Gain3/1, Gain4/1
  Add1/1 -> Gain1/1, Gain2/1, Gain5/1
  Gain1/1 -> Subtract2/1
  Subtract2/1 -> vc/1
  Gain3/1 -> Subtract1/2
  Gain4/1 -> Subtract2/2
  Gain2/1 -> Subtract1/1
  Theta/1 -> Cos1/1, Sin1/1
  Demux/1 -> [vd]
  Demux/2 -> [vq]
  Cos1/1 -> [CosTheta]
  Sin1/1 -> [SinTheta]
  [CosTheta] -> Product1/2
  [CosTheta] -> Product2/2
  [SinTheta] -> Product4/2
  [SinTheta] -> Product3/2
  [vq] -> Product1/1
  [vd] -> Product4/1
  dq/1 -> Demux/1
  Demux/3 -> Terminator/1
